simulink model "tarefa1"  (R2012b)
settings: Solver=ode45  StartTime=0.0  StopTime=4  RelTol=1e-3
values from neighbouring files (symbols this model uses):
  K = 0.02    [Controle_Lab4.m]    (also in Lab8.m = place(A,B,[-10 -12 -2]); Tarefa1.m)
  Kp = Kkp/K    (= 358.333333333)    [Controle_Lab4.m]    (also in Tarefa1.m = 300)
  L = 1.024 - Start    (= 0.024)    [Controle_Lab4.m]    (also in Tarefa1.m = 0.03)
  T = 1.196 - L - Start    (= 0.172)    [Controle_Lab4.m]    (also in Tarefa1.m = 0.18)
settings Model: Creator=11104980  LastModifiedBy=11104980

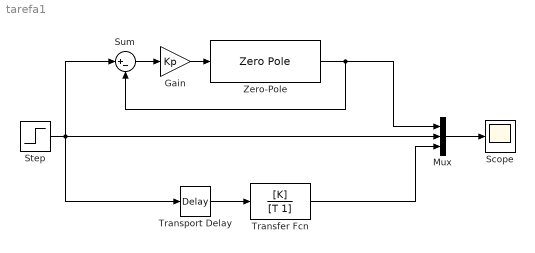
== system tarefa1 ==
  Gain : Gain  Gain=Kp
  Mux : Mux  Inputs=3
  Scope : Scope
      settings: SaveName=y
  Step : Step  SampleTime=0
  Sum : Sum  Inputs=|+-
  Transfer Fcn : TransferFcn  Numerator=[K]  Denominator=[T 1]
  Transport Delay : TransportDelay  DelayTime=L
  Zero-Pole : ZeroPole  Zeros=[]  Poles=[-20 -25 -30]  Gain=[300]
  wires:
  Step/1 -> Transport Delay/1, Sum/1, Mux/2
  Zero-Pole/1 -> Sum/2, Mux/1
  Mux/1 -> Scope/1
  Transport Delay/1 -> Transfer Fcn/1
  Transfer Fcn/1 -> Mux/3
  Sum/1 -> Gain/1
  Gain/1 -> Zero-Pole/1
